simulink model "ProjetoFinal_Controle_1"  (R2022b)
settings: Solver=VariableStepAuto  StartTime=0.0  StopTime=30  RelTol=1e-3
libraries: cstblocks x1
settings Model: Creator=joao_  LastModifiedBy=joao_

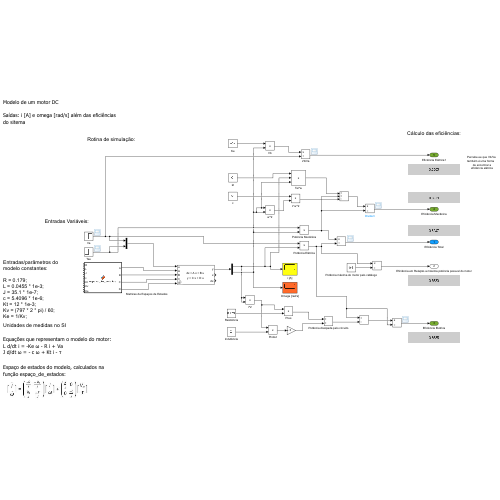
[thumbnail: Simulink's stored preview of the top-level diagram]
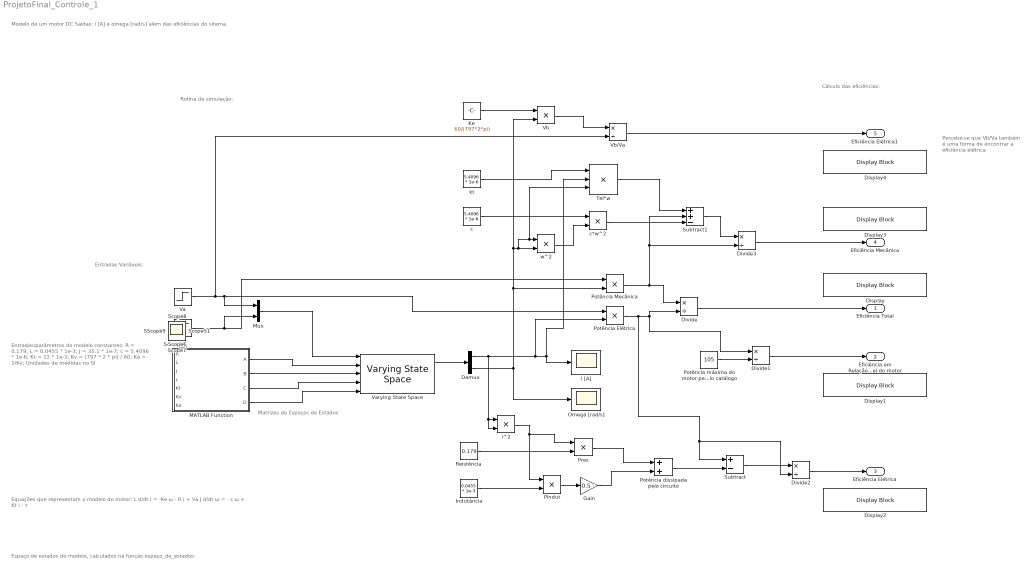
== system ProjetoFinal_Controle_1 ==
  note: Espaço de estados do modelo, calculados na função espaço_de_estados:
  note: Equações que representam o modelo do motor:
      | L d/dt i = -Ke ω - R i + Va
      | J d/dt ω = - c ω + Kt i - τ
  note: Modelo de um motor DC
      |
      | Saídas: i [A] e omega [rad/s] além das eficiências do sitema
  note: Matrizes de Espaços de Estados
  note: Entradas/parâmetros do
      | modelo constantes:
      |
      | R = 0.179;
      | L = 0.0455 * 1e-3;
      | J = 35.1 * 1e-7;
      | c = 5.4096 * 1e-6;
      | Kt = 12 * 1e-3;
      | Kv = (797 * 2 * pi) / 60;
      | Ke = 1/Kv;
      |
      | Unidades de medidas no SI
  note: Entradas Variáveis:
  note: Percebe-se que Vb/Va também é uma forma
      | de encontrar a eficiência elétrica
  note: Rotina de simulação:
  note: Cálculo das eficiências:
  Demux : Demux  Outputs=2
  Display{,1..4} (5 alike) : DisplayBlock  LabelPosition=Hide  Transparency=1
  Divide{,1..3} (4 alike) : Product  Inputs=*/
  Gain : Gain  Gain=0.5
  Indutância : Constant  Value=0.0455 * 1e-3
  Ke : Constant  Value=60/(797*2*pi)
  MATLAB Function : MATLAB Function  TreatAsAtomicUnit=on
  Mux : Mux  Inputs=2
  Omega [rad/s] : Scope
  Pindut : Product
  Potência Elétrica : Product
  Potência Mecânica : Product
  Potência dissipada pelo circuito : Sum
  Potência máxima do motor pelo catálogo : Constant  Value=105
  Pres : Product
  Reistência : Constant  Value=0.179
  Subtract : Sum  Inputs=+-
  Subtract1 : Sum  Inputs=++-
  Tau : Step  Time=10  After=0.091  SampleTime=10
  Tel*w : Product  Inputs=3
  Va : Step  Time=0  Before=10  After=10  SampleTime=0
  Varying State Space : cstblocks/Linear Parameter Varying/Varying State Space  x0=0  xNames=''  OutputX=on  OutputDX=on
  Vb : Product
  Vb/Va : Product  Inputs=*/
  c : Constant  Value=5.4096 * 1e-6
  c*w^2 : Product
  i [A] : Scope
  i^2 : Product
  kt : Constant  Value=5.4096 * 1e-6
  w^2 : Product
  Eficiência Total : Outport
  Eficiência em Relação a máxima potência possvel do motor : Outport  Port=2
  Eficiência Elétrica : Outport  Port=3
  Eficiência Mecânica : Outport  Port=4
  Eficiência Elétrica1 : Outport  Port=5
  Scope{,2..12} (12 alike) : Scope
  wires:
  Va/1 -> Vb/Va/2, Potência Elétrica/1, Mux/1
  Mux/1 -> Varying State Space/1
  Varying State Space/1 -> Demux/1
  Demux/1 -> Tel*w/2, i [A]/1, Potência Elétrica/2, i^2/2, i^2/1
  Demux/2 -> Omega [rad/s]/1, Potência Mecânica/2, Vb/2, w^2/2, Tel*w/3, w^2/1
  MATLAB Function/1(A) -> Varying State Space/2
  MATLAB Function/2(B) -> Varying State Space/3
  MATLAB Function/3(C) -> Varying State Space/4
  MATLAB Function/4(D) -> Varying State Space/5
  Tau/1 -> Potência Mecânica/1, Mux/2
  Potência Mecânica/1 -> Divide3/2, Subtract1/2, Divide/1
  Divide/1 -> Eficiência Total/1
  Potência Elétrica/1 -> Subtract/1, Divide2/2, Divide1/1, Divide/2
  Potência máxima do motor pelo catálogo/1 -> Divide1/2
  Divide1/1 -> Eficiência em Relação a máxima potência possvel do motor/1
  i^2/1 -> Pres/1, Pindut/1
  Reistência/1 -> Pres/2
  Pres/1 -> Potência dissipada pelo circuito/1
  Potência dissipada pelo circuito/1 -> Subtract/2
  Subtract/1 -> Divide2/1
  Divide2/1 -> Eficiência Elétrica/1
  Indutância/1 -> Pindut/2
  Pindut/1 -> Gain/1
  Gain/1 -> Potência dissipada pelo circuito/2
  w^2/1 -> c*w^2/2
  c/1 -> c*w^2/1
  kt/1 -> Tel*w/1
  Divide3/1 -> Eficiência Mecânica/1
  Tel*w/1 -> Subtract1/1
  c*w^2/1 -> Subtract1/3
  Subtract1/1 -> Divide3/1
  Ke/1 -> Vb/1
  Vb/1 -> Vb/Va/1
  Vb/Va/1 -> Eficiência Elétrica1/1

== matlab function ProjetoFinal_Controle_1/MATLAB Function ==
  data: R input; L input; A output; J input; c input; Kt input; Kv input; Ke input; B output; C output; D output
function [A, B, C, D] =  espaco_de_estados(R, L, J, c, Kt, Kv, Ke)



R = 0.179;                  % Ohms
L = 0.0455 * 1e-3;          % mH --> H
J = 35.1 * 1e-7;            % gcm2 --> Kgm2
c = 5.4096 * 1e-6;          % rpm/mNm --> Hz/Nm --> (rad/s)/Nm
Kt = 12 * 1e-3;             % mNm/A --> Nm/A
Kv = (797 * 2 * pi) / 60;   % rpmV/V --> HzV/V --> (rad/s)V/V
Ke = 1/Kv; 


A = [ (-R/L) (-Ke/L);
       (Kt/J) (-c/J)];

B = [ (1/L) 0;
      0 (-1/J)];

C = [1 0;
     0 1];

D = [0 0;
     0 0];

end
